simulink model "PIDTu4_2324"  (Simulink 5.0)
settings: Solver=ode4  StartTime=0.0  StopTime=2  FixedStep=0.01  RelTol=1e-3
libraries: simulink_extras x2
CloseFcn:
  | rtwprivate ssgensfun ModelCloseRequest PID_PI
settings Model: LastModifiedBy=ThinkPad

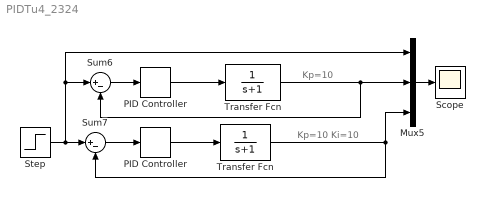
== system PIDTu4_2324 ==
  note: Kp=10 Ki=10
  note: Kp=10
  Mux5 : Mux  Inputs=3
  PID Controller : simulink_extras/Additional Linear/PID Controller  P=10  I=0  D=0
  "PID Controller " : simulink_extras/Additional Linear/PID Controller  P=10  I=10  D=0
  Scope : Scope
      settings: YMin=0  YMax=1.5  SaveName=PIDTu4_24  DataFormat=Array  MaxDataPoints=500000
  Step : Step  Time=0  SampleTime=0
  Sum6 : Sum  Inputs=|+-  SaturateOnIntegerOverflow=on
  Sum7 : Sum  Inputs=|+-  SaturateOnIntegerOverflow=on
  Transfer Fcn : TransferFcn  Denominator=[1 1]
  "Transfer Fcn " : TransferFcn  Denominator=[1 1]
  wires:
  Step/1 -> Sum6/1, Mux5/1, Sum7/1
  Sum6/1 -> PID Controller/1
  PID Controller/1 -> Transfer Fcn/1
  Transfer Fcn/1 -> Sum6/2, Mux5/2
  Mux5/1 -> Scope/1
  Sum7/1 -> "PID Controller "/1
  "PID Controller "/1 -> "Transfer Fcn "/1
  "Transfer Fcn "/1 -> Sum7/2, Mux5/3
